simulink model "ECU"  (R2016b)
settings: Solver=FixedStepAuto  StartTime=0.0  StopTime=inf  FixedStep=ECU.tiSimnTiStep_C  RelTol=1e-3  SampleTimeConstraint=STIndependent  EnableMultiTasking=on
settings Model: Creator=m01wolf  LastModifiedBy=bunver
settings DataIOCC: SaveFormat=StructureWithTime  SaveOutput=off  DSMLogging=off  VisualizeSimOutput=off  SaveTime=off  StateSaveName=Results  SignalLoggingName=Results
settings OptimizationCC: BlockReduction=off  ConditionallyExecuteInputs=off  LifeSpan=inf
settings DebuggingCC: AllowSymbolicDim=off  SFUnexpectedBacktrackingDiag=warning  SFNoUnconditionalDefaultTransitionDiag=warning  SFExecutionAtInitializationDiag=none
settings ModelReferenceCC: ModelReferenceNumInstancesAllowed=Single  PropagateSignalLabelsOutOfModel=off
settings GRTTargetCC: TargetLangStandard=C89/C90 (ANSI)
settings ConfigComp: CovMetricSettings=dw  CovHtmlReporting=on  CovSaveCumulativeToWorkspaceVar=on  CovSaveSingleToWorkspaceVar=on  CovExternalEMLEnable=off

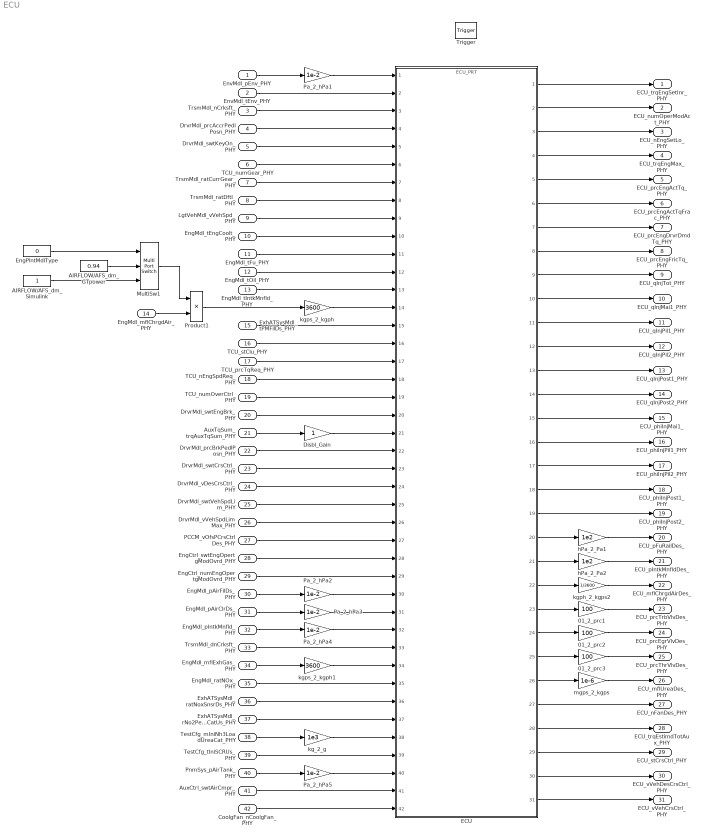
== system ECU ==
  EnvMdl_pEnv_PHY : Inport
  EnvMdl_tEnv_PHY : Inport  Port=2
  TrsmMdl_nCrksft_PHY : Inport  Port=3
  DrvrMdl_prcAccrPedlPosn_PHY : Inport  Port=4
  DrvrMdl_swtKeyOn_PHY : Inport  Port=5
  TCU_numGear_PHY : Inport  Port=6
  TrsmMdl_ratCurrGear_PHY : Inport  Port=7
  TrsmMdl_ratDftl_PHY : Inport  Port=8
  LgtVehMdl_vVehSpd_PHY : Inport  Port=9
  EngMdl_tEngCoolt_PHY : Inport  Port=10
  EngMdl_tFu_PHY : Inport  Port=11
  EngMdl_tOil_PHY : Inport  Port=12
  EngMdl_tIntkMnfld_PHY : Inport  Port=13
  EngMdl_mflChrgdAir_PHY : Inport  Port=14
  ExhATSysMdl_tPMFilDs_PHY : Inport  Port=15
  TCU_stClu_PHY : Inport  Port=16
  TCU_prcTqReq_PHY : Inport  Port=17
  TCU_nEngSpdReq_PHY : Inport  Port=18
  TCU_numOverCtrl_PHY : Inport  Port=19
  DrvrMdl_swtEngBrk_PHY : Inport  Port=20
  AuxTqSum_trqAuxTqSum_PHY : Inport  Port=21
  DrvrMdl_prcBrkPedlPosn_PHY : Inport  Port=22
  DrvrMdl_swtCrsCtrl_PHY : Inport  Port=23
  DrvrMdl_vDesCrsCtrl_PHY : Inport  Port=24
  DrvrMdl_swtVehSpdLim_PHY : Inport  Port=25
  DrvrMdl_vVehSpdLimMax_PHY : Inport  Port=26
  PCCM_vOfsPCrsCtrlDes_PHY : Inport  Port=27
  EngCtrl_swtEngOpertgModOvrd_PHY : Inport  Port=28
  EngCtrl_numEngOpertgModOvrd_PHY : Inport  Port=29
  EngMdl_pAirFilDs_PHY : Inport  Port=30
  EngMdl_pAirClrDs_PHY : Inport  Port=31
  EngMdl_pIntkMnfld_PHY : Inport  Port=32
  TrsmMdl_dnCrksft_PHY : Inport  Port=33
  EngMdl_mflExhGas_PHY : Inport  Port=34
  EngMdl_ratNOx_PHY : Inport  Port=35
  ExhATSysMdl_ratNoxSnsrDs_PHY : Inport  Port=36
  ExhATSysMdl_rNo2PerNoxUreaCatUs_PHY : Inport  Port=37
  TestCfg_mIniNh3LoadUreaCat_PHY : Inport  Port=38
  TestCfg_tIniSCRUs_PHY : Inport  Port=39
  PnmSys_pAirTank_PHY : Inport  Port=40
  AuxCtrl_swtAirCmpr_PHY : Inport  Port=41
  CoolgFan_nCoolgFan_PHY : Inport  Port=42
  Trigger : TriggerPort  TriggerType=function-call  VariantControl=Variant  PortDimensions=1
  01_2_prc1 : Gain  Gain=100
  01_2_prc2 : Gain  Gain=100
  01_2_prc3 : Gain  Gain=100
  AIRFLOW/AFS_dm_GTpower : Constant  Value=0.94  SampleTime=-1
  AIRFLOW/AFS_dm_Simulink : Constant  SampleTime=-1
  Disbl_Gain : Gain
  ECU : ModelReference  ModelNameDialog=ECU_PRT.slxp  ModelReferenceVersion=1.242  CopyOfModelProtected=on
  EngPlntMdlType : Constant  Value=0  SampleTime=-1
  MultiSw1 : MultiPortSwitch  DataPortOrder=Zero-based contiguous  Inputs=2
  Pa_2_hPa{1..5} (5 alike) : Gain  Gain=1e-2
  Product1 : Product  Inputs=**
  hPa_2_Pa1 : Gain  Gain=1e2
  hPa_2_Pa2 : Gain  Gain=1e2
  kg_2_g : Gain  Gain=1e3
  kgph_2_kgps2 : Gain  Gain=1/3600
  kgps_2_kgph : Gain  Gain=3600
  kgps_2_kgph1 : Gain  Gain=3600
  mgps_2_kgps : Gain  Gain=1e-6
  ECU_trqEngSetInr_PHY : Outport
  ECU_numOperModAct_PHY : Outport  Port=2
  ECU_nEngSetLo_PHY : Outport  Port=3
  ECU_trqEngMax_PHY : Outport  Port=4
  ECU_prcEngActTq_PHY : Outport  Port=5
  ECU_prcEngActTqFrac_PHY : Outport  Port=6
  ECU_prcEngDrvrDmdTq_PHY : Outport  Port=7
  ECU_prcEngFricTq_PHY : Outport  Port=8
  ECU_qInjTot_PHY : Outport  Port=9
  ECU_qInjMai1_PHY : Outport  Port=10
  ECU_qInjPil1_PHY : Outport  Port=11
  ECU_qInjPil2_PHY : Outport  Port=12
  ECU_qInjPost1_PHY : Outport  Port=13
  ECU_qInjPost2_PHY : Outport  Port=14
  ECU_phiInjMai1_PHY : Outport  Port=15
  ECU_phiInjPil1_PHY : Outport  Port=16
  ECU_phiInjPil2_PHY : Outport  Port=17
  ECU_phiInjPost1_PHY : Outport  Port=18
  ECU_phiInjPost2_PHY : Outport  Port=19
  ECU_pFuRailDes_PHY : Outport  Port=20
  ECU_pIntkMnfldDes_PHY : Outport  Port=21
  ECU_mflChrgdAirDes_PHY : Outport  Port=22
  ECU_prcTrbVlvDes_PHY : Outport  Port=23
  ECU_prcEgrVlvDes_PHY : Outport  Port=24
  ECU_prcThrVlvDes_PHY : Outport  Port=25
  ECU_mflUreaDes_PHY : Outport  Port=26
  ECU_nFanDes_PHY : Outport  Port=27
  ECU_trqEstimdTotAux_PHY : Outport  Port=28
  ECU_stCrsCtrl_PHY : Outport  Port=29
  ECU_vVehDesCrsCtrl_PHY : Outport  Port=30
  ECU_vVehCrsCtrl_PHY : Outport  Port=31
  wires:
  ECU/1 -> ECU_trqEngSetInr_PHY/1
  ECU/2 -> ECU_numOperModAct_PHY/1
  ECU/3 -> ECU_nEngSetLo_PHY/1
  ECU/4 -> ECU_trqEngMax_PHY/1
  ECU/5 -> ECU_prcEngActTq_PHY/1
  ECU/6 -> ECU_prcEngActTqFrac_PHY/1
  ECU/7 -> ECU_prcEngDrvrDmdTq_PHY/1
  ECU/26 -> mgps_2_kgps/1
  ECU/27 -> ECU_nFanDes_PHY/1
  ECU/15 -> ECU_phiInjMai1_PHY/1
  ECU/14 -> ECU_qInjPost2_PHY/1
  ECU/16 -> ECU_phiInjPil1_PHY/1
  ECU/13 -> ECU_qInjPost1_PHY/1
  ECU/17 -> ECU_phiInjPil2_PHY/1
  ECU/12 -> ECU_qInjPil2_PHY/1
  ECU/18 -> ECU_phiInjPost1_PHY/1
  ECU/11 -> ECU_qInjPil1_PHY/1
  ECU/19 -> ECU_phiInjPost2_PHY/1
  ECU/10 -> ECU_qInjMai1_PHY/1
  ECU/20 -> hPa_2_Pa1/1
  ECU/9 -> ECU_qInjTot_PHY/1
  ECU/23 -> 01_2_prc1/1
  ECU/24 -> 01_2_prc2/1
  ECU/25 -> 01_2_prc3/1
  ECU/8 -> ECU_prcEngFricTq_PHY/1
  Pa_2_hPa1/1 -> ECU/1
  Pa_2_hPa5/1 -> ECU/40
  Pa_2_hPa2/1 -> ECU/30
  Pa_2_hPa3/1 -> ECU/31
  Pa_2_hPa4/1 -> ECU/32
  01_2_prc1/1 -> ECU_prcTrbVlvDes_PHY/1
  01_2_prc2/1 -> ECU_prcEgrVlvDes_PHY/1
  01_2_prc3/1 -> ECU_prcThrVlvDes_PHY/1
  hPa_2_Pa1/1 -> ECU_pFuRailDes_PHY/1
  mgps_2_kgps/1 -> ECU_mflUreaDes_PHY/1
  ECU/29 -> ECU_stCrsCtrl_PHY/1
  ECU/30 -> ECU_vVehDesCrsCtrl_PHY/1
  ECU/31 -> ECU_vVehCrsCtrl_PHY/1
  EnvMdl_pEnv_PHY/1 -> Pa_2_hPa1/1
  EnvMdl_tEnv_PHY/1 -> ECU/2
  TrsmMdl_nCrksft_PHY/1 -> ECU/3
  DrvrMdl_prcAccrPedlPosn_PHY/1 -> ECU/4
  DrvrMdl_swtKeyOn_PHY/1 -> ECU/5
  TCU_numGear_PHY/1 -> ECU/6
  TrsmMdl_ratCurrGear_PHY/1 -> ECU/7
  TrsmMdl_ratDftl_PHY/1 -> ECU/8
  LgtVehMdl_vVehSpd_PHY/1 -> ECU/9
  EngMdl_tEngCoolt_PHY/1 -> ECU/10
  EngMdl_tFu_PHY/1 -> ECU/11
  EngMdl_tOil_PHY/1 -> ECU/12
  EngMdl_tIntkMnfld_PHY/1 -> ECU/13
  TCU_stClu_PHY/1 -> ECU/16
  TCU_prcTqReq_PHY/1 -> ECU/17
  TCU_nEngSpdReq_PHY/1 -> ECU/18
  TCU_numOverCtrl_PHY/1 -> ECU/19
  DrvrMdl_swtEngBrk_PHY/1 -> ECU/20
  DrvrMdl_prcBrkPedlPosn_PHY/1 -> ECU/22
  DrvrMdl_swtCrsCtrl_PHY/1 -> ECU/23
  DrvrMdl_vDesCrsCtrl_PHY/1 -> ECU/24
  DrvrMdl_swtVehSpdLim_PHY/1 -> ECU/25
  DrvrMdl_vVehSpdLimMax_PHY/1 -> ECU/26
  EngMdl_pAirFilDs_PHY/1 -> Pa_2_hPa2/1
  EngMdl_pAirClrDs_PHY/1 -> Pa_2_hPa3/1
  EngMdl_pIntkMnfld_PHY/1 -> Pa_2_hPa4/1
  TrsmMdl_dnCrksft_PHY/1 -> ECU/33
  PnmSys_pAirTank_PHY/1 -> Pa_2_hPa5/1
  ExhATSysMdl_tPMFilDs_PHY/1 -> ECU/15
  PCCM_vOfsPCrsCtrlDes_PHY/1 -> ECU/27
  EngMdl_ratNOx_PHY/1 -> ECU/35
  EngMdl_mflExhGas_PHY/1 -> kgps_2_kgph1/1
  ECU/21 -> hPa_2_Pa2/1
  ECU/22 -> kgph_2_kgps2/1
  hPa_2_Pa2/1 -> ECU_pIntkMnfldDes_PHY/1
  kgph_2_kgps2/1 -> ECU_mflChrgdAirDes_PHY/1
  AuxCtrl_swtAirCmpr_PHY/1 -> ECU/41
  CoolgFan_nCoolgFan_PHY/1 -> ECU/42
  EngCtrl_swtEngOpertgModOvrd_PHY/1 -> ECU/28
  EngCtrl_numEngOpertgModOvrd_PHY/1 -> ECU/29
  kgps_2_kgph1/1 -> ECU/34
  ECU/28 -> ECU_trqEstimdTotAux_PHY/1
  ExhATSysMdl_ratNoxSnsrDs_PHY/1 -> ECU/36
  ExhATSysMdl_rNo2PerNoxUreaCatUs_PHY/1 -> ECU/37
  TestCfg_mIniNh3LoadUreaCat_PHY/1 -> kg_2_g/1
  TestCfg_tIniSCRUs_PHY/1 -> ECU/39
  AuxTqSum_trqAuxTqSum_PHY/1 -> Disbl_Gain/1
  kg_2_g/1 -> ECU/38
  Product1/1 -> kgps_2_kgph/1
  Disbl_Gain/1 -> ECU/21
  EngPlntMdlType/1 -> MultiSw1/1
  AIRFLOW/AFS_dm_Simulink/1 -> MultiSw1/3
  AIRFLOW/AFS_dm_GTpower/1 -> MultiSw1/2
  MultiSw1/1 -> Product1/1
  kgps_2_kgph/1 -> ECU/14
  EngMdl_mflChrgdAir_PHY/1 -> Product1/2
